simulink model "TheSubLayerVersion"  (R2025b)
settings: Solver=ode45  StartTime=0.0  StopTime=0.5  RelTol=1e-3
settings Model: Creator=hp  LastModifiedBy=mulua

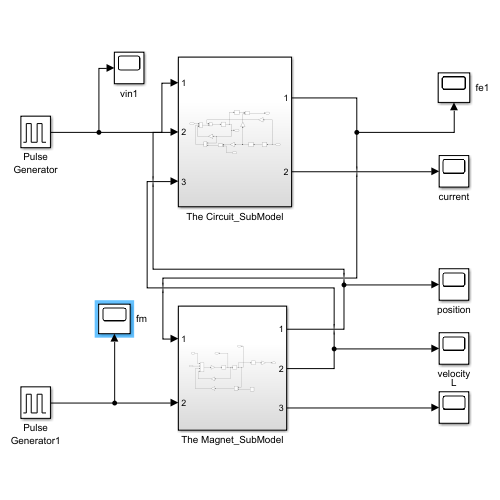
[thumbnail: Simulink's stored preview of the top-level diagram]
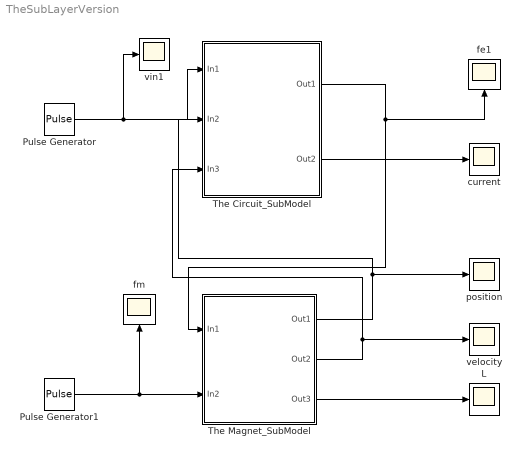
== system TheSubLayerVersion ==
  L : Scope
      settings: ActiveDisplayYMinimum=0.0078185582006970317  ActiveDisplayYMaximum=0.034150500962178268  DataLoggingVariableName=ScopeData3
  Pulse Generator : DiscretePulseGenerator  PulseType=Time based  Amplitude=5  Period=1  PulseWidth=30
  Pulse Generator1 : DiscretePulseGenerator  PulseType=Time based  Amplitude=5  Period=1.0  PulseWidth=15  PhaseDelay=0.15
  The Circuit_SubModel : Subsystem
  The Magnet_SubModel : Subsystem
  current : Scope
      settings: ActiveDisplayYMinimum=-0.066383224764411677  ActiveDisplayYMaximum=0.59744902287970525  DataLoggingVariableName=ScopeData6
  fe1 : Scope
      settings: ActiveDisplayYMinimum=-1.5  ActiveDisplayYMaximum=0
  fm : Scope
      settings: ActiveDisplayYMinimum=-0.62499999999999989  ActiveDisplayYMaximum=5.625  DataLoggingVariableName=ScopeData2
  position : Scope
      settings: ActiveDisplayYMinimum=0.0014912673838802385  ActiveDisplayYMaximum=0.0065136725878086957  DataLoggingVariableName=ScopeData5
  velocity : Scope
      settings: ActiveDisplayYMinimum=-0.37341900147556789  ActiveDisplayYMaximum=0.43149423095817141  DataLoggingVariableName=ScopeData4
  vin1 : Scope
      settings: ActiveDisplayYMinimum=-0.62499999999999989  ActiveDisplayYMaximum=5.625
  wires:
  Pulse Generator/1 -> vin1/1, The Circuit_SubModel/1(In1)
  Pulse Generator1/1 -> The Magnet_SubModel/2(In2), fm/1
  The Circuit_SubModel/1(Out1) -> The Magnet_SubModel/1(In1), fe1/1
  The Magnet_SubModel/3(Out3) -> L/1
  The Magnet_SubModel/2(Out2) -> The Circuit_SubModel/3(In3), velocity/1
  The Magnet_SubModel/1(Out1) -> The Circuit_SubModel/2(In2), position/1
  The Circuit_SubModel/2(Out2) -> current/1

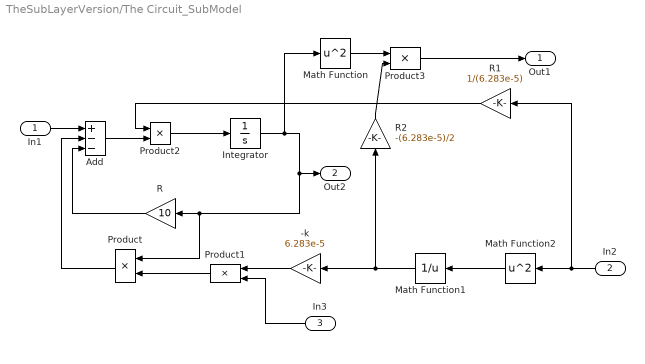
== system TheSubLayerVersion/The Circuit_SubModel ==
  In1 : Inport
  In2 : Inport  Port=2
  In3 : Inport  Port=3
  -k : Gain  Gain=6.283e-5
  Add : Sum  Inputs=+--
  Integrator : Integrator
  Math Function : Math  Operator=square
  Math Function1 : Math  Operator=reciprocal
  Math Function2 : Math  Operator=square
  Product{,1..3} (4 alike) : Product
  R : Gain  Gain=10
  R1 : Gain  Gain=1/(6.283e-5)
  R2 : Gain  Gain=-(6.283e-5)/2
  Out1 : Outport
  Out2 : Outport  Port=2  VectorParamsAs1DForOutWhenUnconnected=off
  wires:
  In1/1 -> Add/1
  Add/1 -> Product2/2
  Product2/1 -> Integrator/1
  Integrator/1 -> Math Function/1, Out2/1, Product/1, R/1
  Product1/1 -> Product/2
  R/1 -> Add/3
  Product/1 -> Add/2
  Math Function/1 -> Product3/1
  R2/1 -> Product3/2
  -k/1 -> Product1/1
  In3/1 -> Product1/2
  Math Function1/1 -> R2/1, -k/1
  Math Function2/1 -> Math Function1/1
  In2/1 -> R1/1, Math Function2/1
  R1/1 -> Product2/1
  Product3/1 -> Out1/1

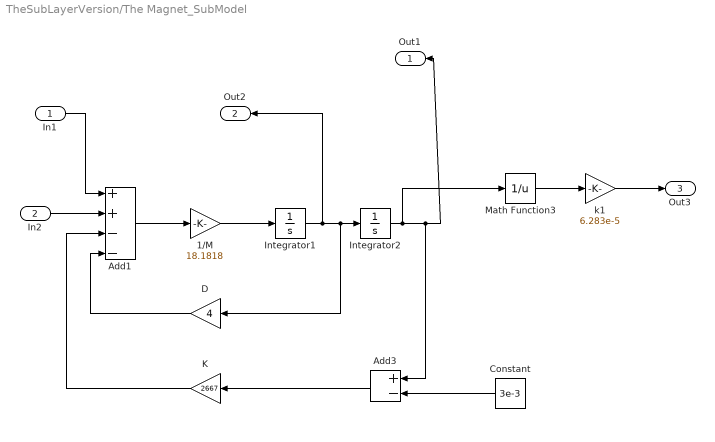
== system TheSubLayerVersion/The Magnet_SubModel ==
  In1 : Inport
  In2 : Inport  Port=2
  1/M : Gain  Gain=18.1818
  Add1 : Sum  Inputs=++--
  Add3 : Sum  Inputs=+-
  Constant : Constant  Value=3e-3
  D : Gain  Gain=4
  Integrator1 : Integrator
  Integrator2 : Integrator  InitialCondition=0.003
  K : Gain  Gain=2667
  Math Function3 : Math  Operator=reciprocal
  k1 : Gain  Gain=6.283e-5
  Out1 : Outport
  Out2 : Outport  Port=2  VectorParamsAs1DForOutWhenUnconnected=off
  Out3 : Outport  Port=3  VectorParamsAs1DForOutWhenUnconnected=off
  wires:
  In2/1 -> Add1/2
  In1/1 -> Add1/1
  Integrator1/1 -> Out2/1, D/1, Integrator2/1
  1/M/1 -> Integrator1/1
  Add3/1 -> K/1
  Constant/1 -> Add3/2
  D/1 -> Add1/4
  K/1 -> Add1/3
  Add1/1 -> 1/M/1
  Integrator2/1 -> Math Function3/1, Add3/1, Out1/1
  k1/1 -> Out3/1
  Math Function3/1 -> k1/1
